simulink model "PolarCinematica"  (R2022a)
settings: Solver=VariableStepAuto  StartTime=0.0  StopTime=Tfinal  RelTol=1e-3
values from neighbouring files (symbols this model uses):
  Tem = Tfinal/length(x)    [Trayectori.m]    (also in lineal.m = 0.001)
undefined symbols (not defined in the file or in its folder): Diferencia, mgd_Polar, mgi_Polar
settings Model: Creator=Shadow  LastModifiedBy=Shadow
settings DebuggingCC: UnconnectedInputMsg=warning  UnconnectedOutputMsg=warning  UnconnectedLineMsg=warning
settings RTWCC: DLArmComputeVersion=19.05

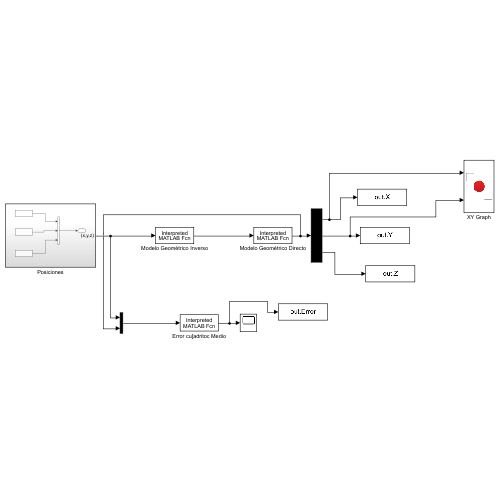
[thumbnail: Simulink's stored preview of the top-level diagram]
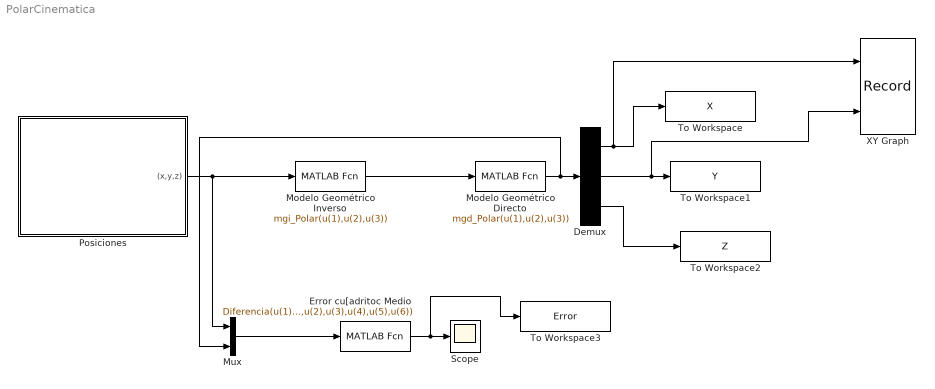
== system PolarCinematica ==
  Demux : Demux  Outputs=3
  Error cu[adritoc Medio : MATLABFcn  MATLABFcn=Diferencia(u(1),u(2),u(3),u(4),u(5),u(6))  OutputDimensions=1
  Modelo Geométrico Directo : MATLABFcn  MATLABFcn=mgd_Polar(u(1),u(2),u(3))  OutputDimensions=3
  Modelo Geométrico Inverso : MATLABFcn  MATLABFcn=mgi_Polar(u(1),u(2),u(3))  OutputDimensions=3
  Mux : Mux  Inputs=2
  Posiciones : Subsystem
  Scope : Scope
  To Workspace : ToWorkspace  VariableName=X
  To Workspace1 : ToWorkspace  VariableName=Y
  To Workspace2 : ToWorkspace  VariableName=Z
  To Workspace3 : ToWorkspace  VariableName=Error
  XY Graph : Record  FileSettingsInternal="{\"entries\":[{\"content\":{\"excelSettings\":{\"content\":{},\"type\":\"Streamout.ExcelSettings\"}},\"type\":\"Streamout.FileSettingStorage\",\"uuid\":\"f9274f99-a235-4885-9da2-32b7dcb45e0b\"}],\"packageUris\":[\"http://schema.mathworks.com/mf0/streamout_blocks/R2020a\"],\"version\":\"1.0\"}"  Layout=[1 1]  SignalsInternal="{\"entries\":[{\"content\":{\"signals\":[{\"content\":{\"blockPath\":[\"PolarCinematica/XY Graph\"],\"channel\":[],\"dimensions\":[1],\"domain\":\"PolarCinematica/XY Graph\",\"lineColor\":\"#a2142f\",\"plots\":[1],\"port\":1,\"sid\":[\"\"],\"signalID\":78,\"signalName\":\"Demux:1\"},\"type\":\"RecordBlkView.Signal\",\"uuid\":\"8cb81a2b-5ffc-4bf8-93c4-22765202057e\"},{\"content\":{\"blockPath\":[\"PolarCinematica/XY Graph\"],\"channel\":[],\"dimensions\":[1],\"domain\":\"PolarCinematica/XY Graph\",\"lineColor\":\"#139fff\",\"plots\":[1],\"port\":2,\"sid\":[\"\"],\"signalID\":82,\"signalName\":\"Demux:2\"},\"type\":\"RecordBlkView.Signal\",\"uuid\":\"50062af5-6a11-4fc5-af7f-56daddc45090\"}]},\"type\":\"RecordBlkView.InputSignals\",\"uuid\":\"b85599bc-bccc-4398-b62e-5b5cdddf0632\"}],\"packageUris\":[\"http://schema.mathworks.com/mf0/streamout_blocks/R2020a\"],\"version\":\"1.0\"}"  VisualizationBindings="{\"xyplotplugin\":{\"info\":[{\"series\":[{\"bindingParametersList\":[{\"parameter\":\"X-Axis\",\"signalID\":78,\"signalName\":\"Demux:1\"},{\"parameter\":\"Y-Axis\",\"signalID\":82,\"signalName\":\"Demux:2\"}],\"seriesID\":1531}],\"subplotID\":1}]}}"  CompatibilityTag=XY
  wires:
  Demux/2 -> XY Graph/2, To Workspace1/1
  Demux/3 -> To Workspace2/1
  Modelo Geométrico Inverso/1 -> Modelo Geométrico Directo/1
  Posiciones/1((x,y,z)) -> Mux/1, Modelo Geométrico Inverso/1
  Demux/1 -> To Workspace/1, XY Graph/1
  Mux/1 -> Error cu[adritoc Medio/1
  Modelo Geométrico Directo/1 -> Mux/2, Demux/1
  Error cu[adritoc Medio/1 -> To Workspace3/1, Scope/1

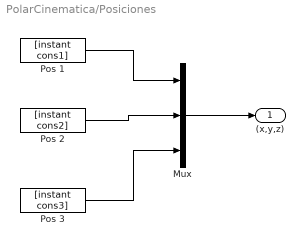
== system PolarCinematica/Posiciones ==
  Mux : Mux  Inputs=3
  Pos 1 : FromWorkspace  VariableName=[instant cons1]  SampleTime=Tem
  Pos 2 : FromWorkspace  VariableName=[instant cons2]  SampleTime=Tem
  Pos 3 : FromWorkspace  VariableName=[instant cons3]  SampleTime=Tem
  (x,y,z) : Outport
  wires:
  Pos 3/1 -> Mux/3
  Pos 1/1 -> Mux/1
  Pos 2/1 -> Mux/2
  Mux/1 -> (x,y,z)/1
